simulink model "motor_cc"  (R2016b)
settings: Solver=VariableStepAuto  StartTime=1  StopTime=100  RelTol=1e-3
settings Model: Creator=groscoe  LastModifiedBy=groscoe

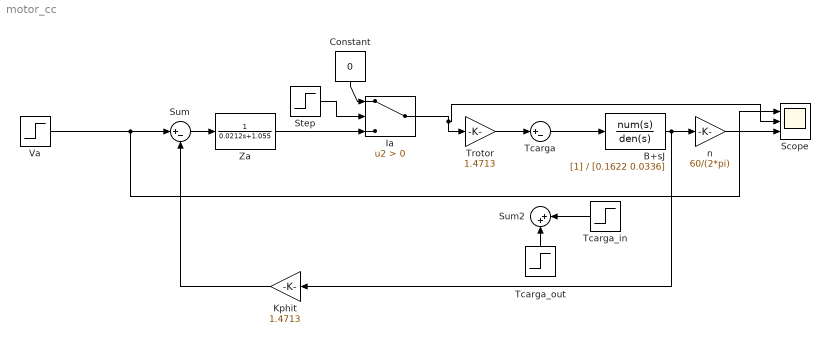
== system motor_cc ==
  "B+sJ " : TransferFcn  Denominator=[0.1622 0.0336]
  Constant : Constant  Value=0
  Ia : Switch  Criteria=u2 > Threshold
  Kphit : Gain  Gain=1.4713
  Scope : Scope  NumInputPorts=3
  Step : Step  Time=10  Before=-1  After=-1  SampleTime=0
  Sum : Sum  Inputs=|+-
  Sum2 : Sum  Inputs=|++
  "Tcarga " : Sum  Inputs=|+-
  Tcarga_in : Step  Time=3  After=18.58  SampleTime=0
  Tcarga_out : Step  Time=5  After=-18.58  SampleTime=0
  Trotor : Gain  Gain=1.4713
  Va : Step  Time=0  After=42  SampleTime=0
  Za : TransferFcn  Denominator=[0.0212 1.055]
  n : Gain  Gain=60/(2*pi)
  wires:
  Va/1 -> Scope/1, Sum/1
  Sum/1 -> Za/1
  Ia/1 -> Scope/2, Trotor/1
  Kphit/1 -> Sum/2
  "B+sJ "/1 -> Kphit/1, n/1
  Trotor/1 -> "Tcarga "/1
  "Tcarga "/1 -> "B+sJ "/1
  Tcarga_in/1 -> Sum2/2
  Tcarga_out/1 -> Sum2/1
  Za/1 -> Ia/3
  Step/1 -> Ia/2
  Constant/1 -> Ia/1
  n/1 -> Scope/3
